simulink model "Lab12_Task2"  (R2016a)
settings: Solver=VariableStepAuto  StartTime=0.0  StopTime=10.0  RelTol=1e-3
settings Model: Creator=DELL  LastModifiedBy=DELL

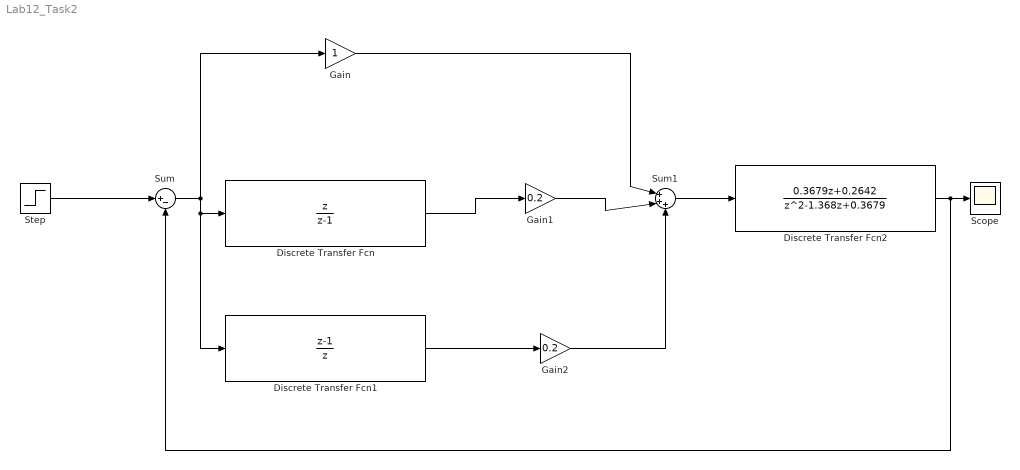
== system Lab12_Task2 ==
  Discrete Transfer Fcn : DiscreteTransferFcn  Numerator=[1 0]  Denominator=[1 -1]  InitialStates=1
  Discrete Transfer Fcn1 : DiscreteTransferFcn  Numerator=[1 -1]  Denominator=[1 0]
  Discrete Transfer Fcn2 : DiscreteTransferFcn  Numerator=[0.3679 0.2642]  Denominator=[1 -1.368 0.3679]  InitialStates=1
  Gain : Gain
  Gain1 : Gain  Gain=0.2
  Gain2 : Gain  Gain=0.2
  Scope : Scope
  Step : Step  SampleTime=1
  Sum : Sum  Inputs=|+-
  Sum1 : Sum  Inputs=|+++
  wires:
  Step/1 -> Sum/1
  Sum/1 -> Discrete Transfer Fcn1/1, Discrete Transfer Fcn/1, Gain/1
  Gain1/1 -> Sum1/2
  Gain2/1 -> Sum1/3
  Gain/1 -> Sum1/1
  Sum1/1 -> Discrete Transfer Fcn2/1
  Discrete Transfer Fcn1/1 -> Gain2/1
  Discrete Transfer Fcn/1 -> Gain1/1
  Discrete Transfer Fcn2/1 -> Sum/2, Scope/1
